simulink model "vincadorM"  (R2018b)
settings: Solver=VariableStepAuto  StartTime=0.0  StopTime=Tsimul  MaxStep=maxstep  RelTol=1e-3
values from neighbouring files (symbols this model uses):
  delay1 = Tencoder*(TpulseFraction)    (= 6.28318530718e-05)    [vincadorS.m]
  delay2 = Tencoder*(TpulseFraction/2)    (= 3.14159265359e-05)    [vincadorS.m]
  maxstep = TSampler/10    (= 2e-09)    [vincadorS.m]
  pulsosPorVolta = 500    [vincadorS.m]
  Tencoder = Trotacao/pulsosPorVolta    (= 0.000251327412287)    [vincadorS.m]
  TpulseFraction = 0.25    [vincadorS.m]
  Trotacao = 1/rps    (= 0.125663706144)    [vincadorS.m]
  TSampler = 1/fSampler    (= 2e-08)    [vincadorS.m]
libraries: simulink x12, simulink_extras x4
settings Model: Creator=mauri  LastModifiedBy=mauri

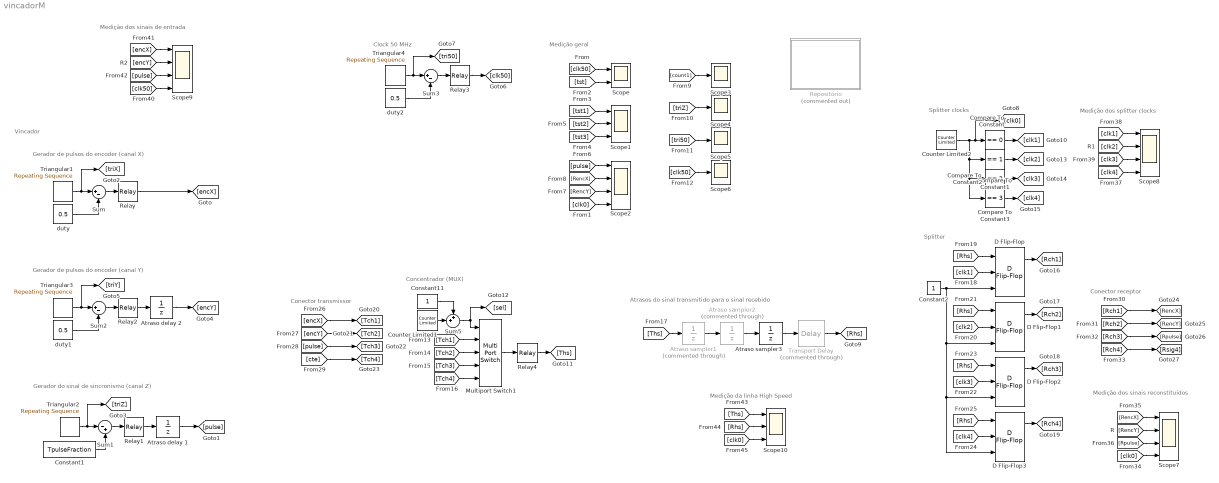
== system vincadorM ==
  note: Concentrador (MUX)
  note: Vincador
  note: Medição da linha High Speed
  note: Medição dos sinais
      | reconstituídos
  note: Conector transmissor
  note: Splitter
  note: Splitter clocks
  note: Atrasos do sinal transmitido para o sinal recebido
  note: Medição geral
  note: Clock 50 MHz
  note: Gerador do sinal de sincronismo (canal Z)
  note: Gerador de pulsos do encoder (canal X)
  note: Gerador de pulsos do encoder (canal Y)
  note: Conector receptor
  note: Medição dos splitter clocks
  note: Medição dos sinais de entrada
  Atraso sampler1 : UnitDelay  Commented=through  SampleTime=TSampler
  Atraso sampler2 : UnitDelay  Commented=through  SampleTime=TSampler
  Atraso sampler3 : UnitDelay  SampleTime=maxstep*5
  Atraso delay 1 : UnitDelay  SampleTime=delay1
  Atraso delay 2 : UnitDelay  SampleTime=delay2
  Compare To Constant : simulink/Logic and Bit Operations/Compare To Constant  relop===  const=0  OutDataTypeStr=boolean
  Compare To Constant1 : simulink/Logic and Bit Operations/Compare To Constant  relop===  const=1  OutDataTypeStr=boolean
  Compare To Constant2 : simulink/Logic and Bit Operations/Compare To Constant  relop===  const=2  OutDataTypeStr=boolean
  Compare To Constant3 : simulink/Logic and Bit Operations/Compare To Constant  relop===  const=3  OutDataTypeStr=boolean
  Constant1 : Constant  Value=TpulseFraction
  Constant11 : Constant
  Constant2 : Constant
  Counter Limited1 : simulink/Sources/Counter Limited  uplimit=3  tsamp=TSampler
  Counter Limited2 : simulink/Sources/Counter Limited  uplimit=3  tsamp=TSampler
  D Flip-Flop{,1..3} (4 alike) : simulink_extras/Flip Flops/D Flip-Flop
      settings: SourceProductName=Simulink
  Multiport Switch1 : MultiPortSwitch  Inputs=4  DiagnosticForDefault=None
  Relay{,1..3} (4 alike) : Relay
  Relay4 : Relay  OnSwitchValue=eps+0.5  OffSwitchValue=eps+0.5  OutDataTypeStr=boolean
  Repositório : Subsystem  Commented=on
  Scope : Scope  NumInputPorts=2
  Scope1 : Scope  NumInputPorts=3
  Scope10 : Scope  NumInputPorts=3
  Scope{2,7..9} (4 alike) : Scope  NumInputPorts=4
  Scope{3..6} (4 alike) : Scope
  Sum : Sum  Inputs=|+-
  Sum1 : Sum  Inputs=|-+
  Sum2 : Sum  Inputs=|+-
  Sum3 : Sum  Inputs=|+-
  Sum5 : Sum  Inputs=++|
  Transport Delay : TransportDelay  Commented=through  DelayTime=maxstep*5
  Triangular1 : simulink/Sources/Repeating Sequence  rep_seq_t=[0 Tencoder]  rep_seq_y=[0 1]
  Triangular2 : simulink/Sources/Repeating Sequence  rep_seq_t=[0 Trotacao]  rep_seq_y=[0 pulsosPorVolta]
  Triangular3 : simulink/Sources/Repeating Sequence  rep_seq_t=[0 Tencoder]  rep_seq_y=[0 1]
  Triangular4 : simulink/Sources/Repeating Sequence  rep_seq_t=[0 TSampler]  rep_seq_y=[0 1]
  duty : Constant  Value=0.5
  duty1 : Constant  Value=0.5
  duty2 : Constant  Value=0.5
  wires:
  Sum/1 -> Relay/1
  Triangular1/1 -> [triX], Sum/1
  duty/1 -> Sum/2
  Constant1/1 -> Sum1/2
  Triangular2/1 -> [triZ], Sum1/1
  Sum1/1 -> Relay1/1
  [clk50] -> Scope/1
  Relay/1 -> [encX]
  Relay1/1 -> Atraso delay 1/1
  Atraso delay 1/1 -> [pulse]
  Relay2/1 -> Atraso delay 2/1
  duty1/1 -> Sum2/2
  Triangular3/1 -> Sum2/1, [triY]
  Sum2/1 -> Relay2/1
  Atraso delay 2/1 -> [encY]
  [tst] -> Scope/2
  Triangular4/1 -> [tri50], Sum3/1
  duty2/1 -> Sum3/2
  Sum3/1 -> Relay3/1
  Relay3/1 -> [clk50]
  [tst2] -> Scope1/2
  [tst3] -> Scope1/3
  [tst1] -> Scope1/1
  [pulse] -> Scope2/1
  [RencY] -> Scope2/3
  [RencX] -> Scope2/2
  [clk0] -> Scope2/4
  [count1] -> Scope3/1
  [triZ] -> Scope4/1
  [tri50] -> Scope5/1
  [clk50] -> Scope6/1
  Sum5/1 -> Multiport Switch1/1, [sel]
  Constant11/1 -> Sum5/1
  Counter Limited1/1 -> Sum5/2
  [Tch1] -> Multiport Switch1/2
  [Tch2] -> Multiport Switch1/3
  [Tch3] -> Multiport Switch1/4
  [Tch4] -> Multiport Switch1/5
  Atraso sampler2/1 -> Atraso sampler3/1
  Atraso sampler1/1 -> Atraso sampler2/1
  [Ths] -> Atraso sampler1/1
  Atraso sampler3/1 -> Transport Delay/1
  Compare To Constant/1 -> [clk1]
  Counter Limited2/1 -> Compare To Constant1/1, Compare To Constant2/1, Compare To Constant3/1, [clk0], Compare To Constant/1
  Compare To Constant1/1 -> [clk2]
  Compare To Constant2/1 -> [clk3]
  Compare To Constant3/1 -> [clk4]
  [Rhs] -> D Flip-Flop/1
  [clk1] -> D Flip-Flop/2
  D Flip-Flop/1 -> [Rch1]
  D Flip-Flop1/1 -> [Rch2]
  [clk2] -> D Flip-Flop1/2
  [Rhs] -> D Flip-Flop1/1
  [Rhs] -> D Flip-Flop2/1
  [clk3] -> D Flip-Flop2/2
  D Flip-Flop2/1 -> [Rch3]
  D Flip-Flop3/1 -> [Rch4]
  [clk4] -> D Flip-Flop3/2
  [Rhs] -> D Flip-Flop3/1
  Transport Delay/1 -> [Rhs]
  [encX] -> [Tch1]
  [encY] -> [Tch2]
  [pulse] -> [Tch3]
  [cte] -> [Tch4]
  [Rch4] -> [Rsig4]
  [Rch3] -> [Rpulse]
  [Rch2] -> [RencY]
  [Rch1] -> [RencX]
  [clk0] -> Scope7/4
  [RencY] -> Scope7/2
  [Rpulse] -> Scope7/3
  [RencX] -> Scope7/1
  [clk1] -> Scope8/1
  [clk3] -> Scope8/3
  [clk2] -> Scope8/2
  [clk4] -> Scope8/4
  [clk50] -> Scope9/4
  [encY] -> Scope9/2
  [pulse] -> Scope9/3
  [encX] -> Scope9/1
  [Ths] -> Scope10/1
  [Rhs] -> Scope10/2
  [clk0] -> Scope10/3
  Multiport Switch1/1 -> Relay4/1
  Relay4/1 -> [Ths]
  Constant2/1 -> D Flip-Flop/3, D Flip-Flop1/3, D Flip-Flop2/3, D Flip-Flop3/3

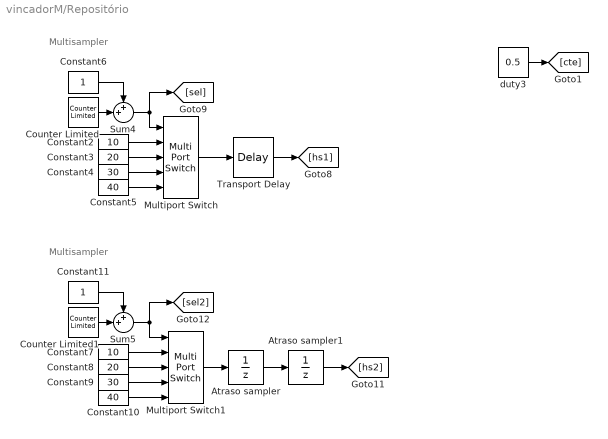
== system vincadorM/Repositório ==
  note: Multisampler
  note: Multisampler
  Atraso sampler : UnitDelay  SampleTime=TSampler
  Atraso sampler1 : UnitDelay  SampleTime=TSampler
  Constant10 : Constant  Value=40
  Constant11 : Constant
  Constant2 : Constant  Value=10
  Constant3 : Constant  Value=20
  Constant4 : Constant  Value=30
  Constant5 : Constant  Value=40
  Constant6 : Constant
  Constant7 : Constant  Value=10
  Constant8 : Constant  Value=20
  Constant9 : Constant  Value=30
  Counter Limited : simulink/Sources/Counter Limited  uplimit=3  tsamp=TSampler
  Counter Limited1 : simulink/Sources/Counter Limited  uplimit=3  tsamp=TSampler
  Multiport Switch : MultiPortSwitch  Inputs=4  DiagnosticForDefault=None
  Multiport Switch1 : MultiPortSwitch  Inputs=4  DiagnosticForDefault=None
  Sum4 : Sum  Inputs=++|
  Sum5 : Sum  Inputs=++|
  Transport Delay : TransportDelay  DelayTime=TSampler*2
  duty3 : Constant  Value=0.5
  wires:
  Constant6/1 -> Sum4/1
  Constant5/1 -> Multiport Switch/5
  Constant4/1 -> Multiport Switch/4
  Sum4/1 -> [sel], Multiport Switch/1
  Constant2/1 -> Multiport Switch/2
  Constant3/1 -> Multiport Switch/3
  Transport Delay/1 -> [hs1]
  Counter Limited/1 -> Sum4/2
  Multiport Switch/1 -> Transport Delay/1
  Multiport Switch1/1 -> Atraso sampler/1
  Atraso sampler/1 -> Atraso sampler1/1
  Constant7/1 -> Multiport Switch1/2
  Constant10/1 -> Multiport Switch1/5
  Counter Limited1/1 -> Sum5/2
  Constant8/1 -> Multiport Switch1/3
  Constant9/1 -> Multiport Switch1/4
  Constant11/1 -> Sum5/1
  Atraso sampler1/1 -> [hs2]
  Sum5/1 -> Multiport Switch1/1, [sel2]
  duty3/1 -> [cte]
